simulink model "kuramoto_notFlashing"  (Simulink 7.8)
settings: Solver=ode45  StartTime=0.0  StopTime=10.0  RelTol=1e-3
undefined symbols (not defined in the file): K, N, omega, rho0
Description:
  | Kuramoto oscillator model
  | copy Jose Rivera
  | chepeadan@gmail.com
settings Model: Creator=chepeadan  LastModifiedBy=trommsdorff
settings DebuggingCC: FcnCallInpInsideContextMsg=Use local settings  StrictBusMsg=Warning

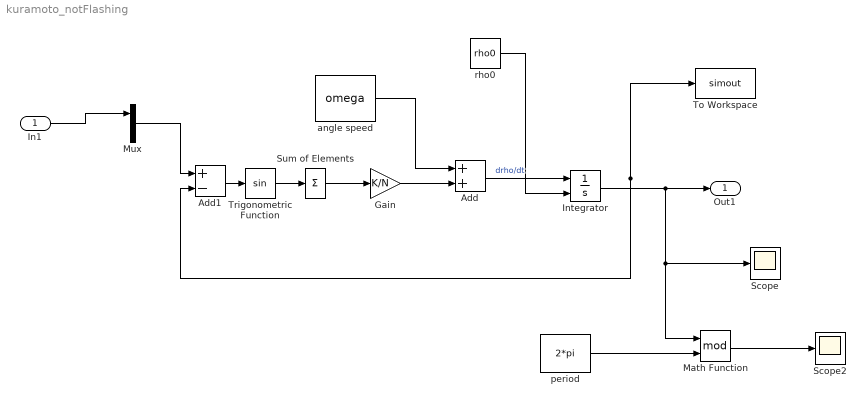
== system kuramoto_notFlashing ==
  In1 : Inport
  Add : Sum
  Add1 : Sum  Inputs=+-
  Gain : Gain  Gain=K/N
  Integrator : Integrator  InitialConditionSource=external
  Math Function : Math  Operator=mod  SaturateOnIntegerOverflow=on
  Mux : Mux  Inputs=2
  Scope : Scope
  Scope2 : Scope
      settings: SaveName=ScopeData2
  Sum of Elements : Sum  Inputs=+
  To Workspace : ToWorkspace  VariableName=simout  SampleTime=-1  SaveFormat=Structure With Time
  Trigonometric Function : Trigonometry
  angle speed : Constant  Value=omega
  period : Constant  Value=2*pi
  rho0 : Constant  Value=rho0
  Out1 : Outport
  wires:
  In1/1 -> Mux/1
  Mux/1 -> Add1/1
  Add1/1 -> Trigonometric Function/1
  angle speed/1 -> Add/1
  Gain/1 -> Add/2
  Add/1 -> Integrator/1  "drho/dt"
  Trigonometric Function/1 -> Sum of Elements/1
  Sum of Elements/1 -> Gain/1
  rho0/1 -> Integrator/2
  period/1 -> Math Function/2
  Math Function/1 -> Scope2/1
  Integrator/1 -> Add1/2, To Workspace/1, Out1/1, Scope/1, Math Function/1
